simulink model "mvdc_state_estimation"  (R2018b)
settings: configuration reference "Active" (kept outside this file)
undefined symbols (not defined in the file): l_front_m, l_rear_m, P_MLOC_MaxWheelslip_perc, P_MLOC_MaxWheelslipangle_rad, P_MLOC_MinWheelslip_perc, P_MLOC_MinWheelslipangle_rad, P_VDC_ActivateSensorFusion, P_VDC_CurvatureEstimateMax_radpm, P_VDC_CurvatureEstimationMode, P_VDC_LowPassRawSens, P_VDC_LowPassT1Curvature, P_VDC_MinVelSlipCalc_mps, P_VDC_SEResetSamples, tS, TUMStateEstimationState, tw_front_m, tw_rear_m, tyreradius_front_m, tyreradius_rear_m
libraries: simulink x19, misc x3
settings Model: DataDictionary=mvdc_state_estimation.sldd  Creator=wischnewski  LastModifiedBy=ge34qer

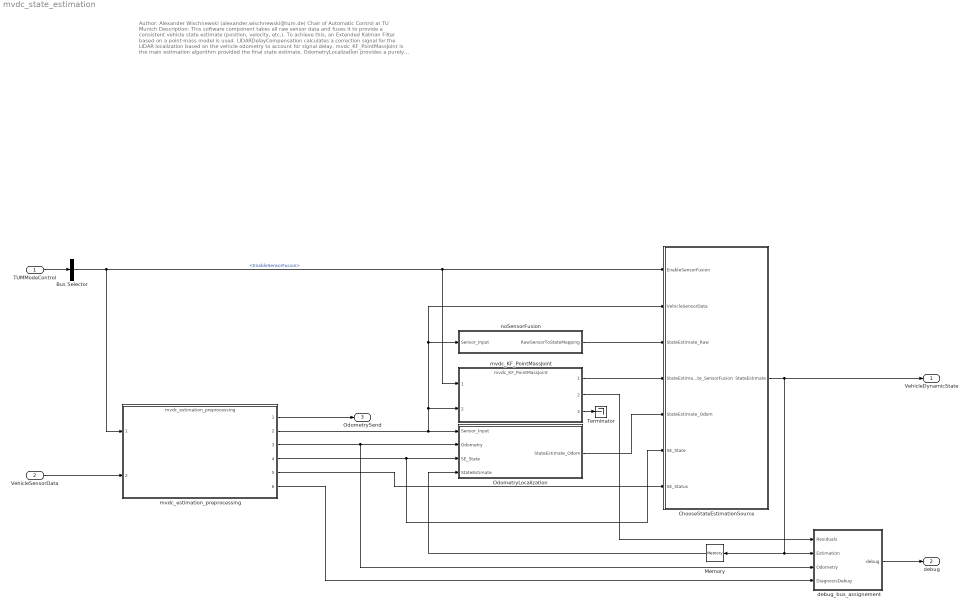
== system mvdc_state_estimation ==
  note: Author: Alexander Wischnewski (alexander.wischnewski@tum.de)
      | Chair of Automatic Control at TU Munich
      |
      | Description: This software component takes all raw sensor data and fuses it to provide a consistent vehicle state estimate (position, velocity, etc.).
      | To achieve this, an Extended Kalman Filter based on a point-mass model is used.
      |
      | LIDARDelayCompensation calculates a correction signal for the LIDAR localization based on the vehicle odometry to account for signal delay.
      |
      | mvdc_KF_PointMassJoint is the main estimation algorithm provided the final state estimate.
      |
      | OdometryLocalization provides a purely odometry based localization based on the last valid position.
      |
      | noSensorFusion provides a bypass solution to the estimator and is used while EnableSensorFusion is not set.
      |
      | mvdc_estimation_preprocessing applies diagnostics on the sensors and generates odometry information.
      |
      | Finally, the debug_bus_assignment forms the debug data.
      |
      | Inputs:
      | TUMModeControl Enable bits which activate the Kalman Filter
      | VehicleSensorData Raw sensor data
      |
      | Outputs:
      | VehicleDynamicState Estimate of the vehicle dynamic state (best available)
      | debug debug data for logging
      | VisualLocSend Data which is send to the LIDAR localization algorithm
  TUMModeControl : Inport  OutDataTypeStr=Bus: TUMModeControl  PortDimensions=1  BusOutputAsStruct=on
  VehicleSensorData : Inport  Port=2  OutDataTypeStr=Bus: VehicleSensorData
  Bus Selector : BusSelector  OutputSignals=EnableSensorFusion
  ChooseStateEstimationSource : Subsystem
  Memory : Memory
  OdometryLocalization : Subsystem
  Terminator : Terminator
  debug_bus_assignement : Subsystem
  mvdc_KF_PointMassJoint : ModelReference  ModelNameDialog=mvdc_KF_PointMassJoint.slx  SimulationMode=Normal  ModelReferenceVersion=1.174
  mvdc_estimation_preprocessing : ModelReference  ModelNameDialog=mvdc_estimation_preprocessing  SimulationMode=Normal  ModelReferenceVersion=1.392
  noSensorFusion : Subsystem
  VehicleDynamicState : Outport  OutDataTypeStr=Bus: VehicleDynamicState
  debug : Outport  Port=2  OutDataTypeStr=Bus: mvdc_state_estimation_debug  PortDimensions=1
  OdometrySend : Outport  Port=3  OutDataTypeStr=Bus: VisualLoc_Send  BusOutputAsStruct=on
  wires:
  mvdc_KF_PointMassJoint/1 -> ChooseStateEstimationSource/4(StateEstimate_SensorFusion)
  Bus Selector/1 -> mvdc_KF_PointMassJoint/1, ChooseStateEstimationSource/1(EnableSensorFusion), mvdc_estimation_preprocessing/1  "<EnableSensorFusion>"
  mvdc_estimation_preprocessing/4 -> ChooseStateEstimationSource/6(SE_State), OdometryLocalization/3(SE_State)
  VehicleSensorData/1 -> mvdc_estimation_preprocessing/2
  mvdc_estimation_preprocessing/2 -> ChooseStateEstimationSource/2(VehicleSensorData), noSensorFusion/1(Sensor_Input), mvdc_KF_PointMassJoint/2, OdometryLocalization/1(Sensor_Input)
  mvdc_estimation_preprocessing/1 -> OdometrySend/1
  ChooseStateEstimationSource/1(StateEstimate) -> Memory/1, debug_bus_assignement/2(Estimation), VehicleDynamicState/1
  mvdc_estimation_preprocessing/3 -> debug_bus_assignement/3(Odometry), OdometryLocalization/2(Odometry)
  OdometryLocalization/1(StateEstimate_Odom) -> ChooseStateEstimationSource/5(StateEstimate_Odom)
  noSensorFusion/1(RawSensorToStateMapping) -> ChooseStateEstimationSource/3(StateEstimate_Raw)
  Memory/1 -> OdometryLocalization/4(StateEstimate)
  debug_bus_assignement/1(debug) -> debug/1
  mvdc_estimation_preprocessing/5 -> ChooseStateEstimationSource/7(SE_Status)
  mvdc_KF_PointMassJoint/2 -> debug_bus_assignement/1(Residuals)
  mvdc_KF_PointMassJoint/3 -> Terminator/1
  TUMModeControl/1 -> Bus Selector/1
  mvdc_estimation_preprocessing/6 -> debug_bus_assignement/4(DiagnosisDebug)

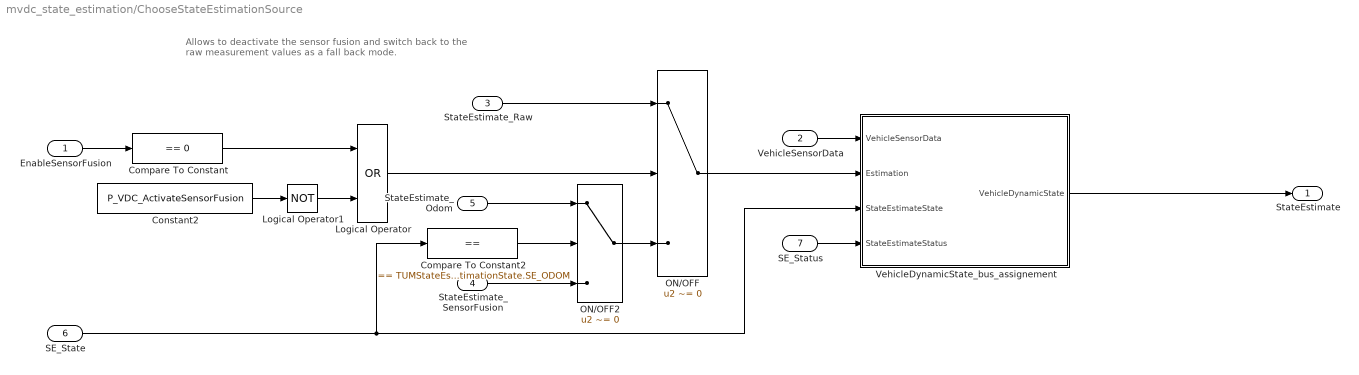
== system mvdc_state_estimation/ChooseStateEstimationSource ==
  note: Allows to deactivate the sensor fusion and switch
      | back to the raw measurement values as a fall back mode.
  EnableSensorFusion : Inport
  VehicleSensorData : Inport  Port=2
  StateEstimate_Raw : Inport  Port=3
  StateEstimate_SensorFusion : Inport  Port=4
  StateEstimate_Odom : Inport  Port=5
  SE_State : Inport  Port=6
  SE_Status : Inport  Port=7
  Compare To Constant : simulink/Logic and Bit Operations/Compare To Constant  relop===  const=0  OutDataTypeStr=boolean
  Compare To Constant2 : simulink/Logic and Bit Operations/Compare To Constant  relop===  const=TUMStateEstimationState.SE_ODOM  OutDataTypeStr=boolean
  Constant2 : Constant  Value=P_VDC_ActivateSensorFusion
  Logical Operator : Logic  Operator=OR  AllPortsSameDT=off  OutDataTypeStr=boolean
  Logical Operator1 : Logic  Operator=NOT  AllPortsSameDT=off  OutDataTypeStr=boolean
  ON/OFF : Switch  Criteria=u2 ~= 0
  ON/OFF2 : Switch  Criteria=u2 ~= 0
  VehicleDynamicState_bus_assignement : Subsystem
  StateEstimate : Outport
  wires:
  StateEstimate_Raw/1 -> ON/OFF/1
  Logical Operator/1 -> ON/OFF/2
  Compare To Constant/1 -> Logical Operator/1
  EnableSensorFusion/1 -> Compare To Constant/1
  SE_State/1 -> VehicleDynamicState_bus_assignement/3(StateEstimateState), Compare To Constant2/1
  ON/OFF/1 -> VehicleDynamicState_bus_assignement/2(Estimation)
  VehicleSensorData/1 -> VehicleDynamicState_bus_assignement/1(VehicleSensorData)
  SE_Status/1 -> VehicleDynamicState_bus_assignement/4(StateEstimateStatus)
  VehicleDynamicState_bus_assignement/1(VehicleDynamicState) -> StateEstimate/1
  ON/OFF2/1 -> ON/OFF/3
  Compare To Constant2/1 -> ON/OFF2/2
  StateEstimate_Odom/1 -> ON/OFF2/1
  StateEstimate_SensorFusion/1 -> ON/OFF2/3
  Constant2/1 -> Logical Operator1/1
  Logical Operator1/1 -> Logical Operator/2

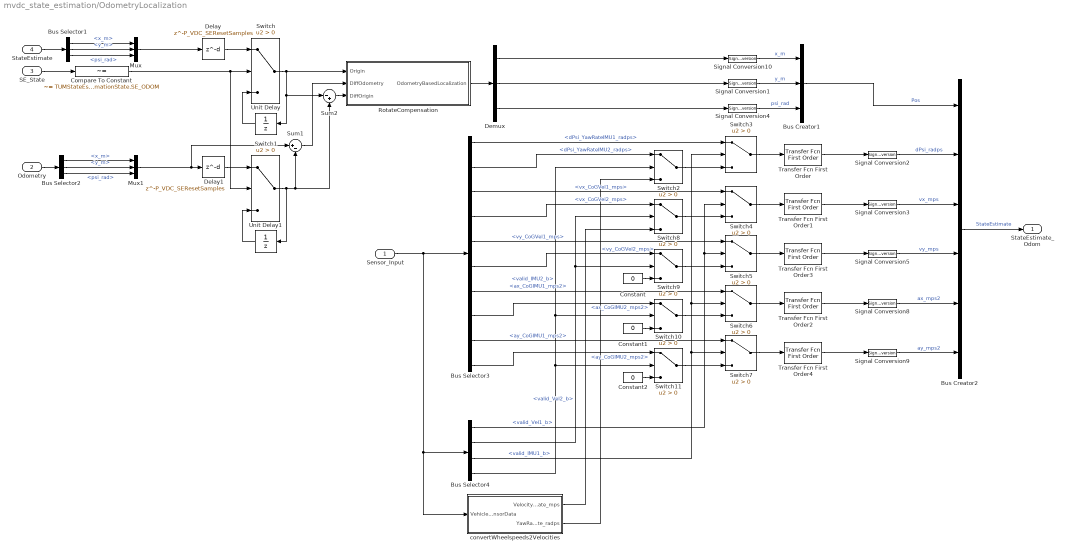
== system mvdc_state_estimation/OdometryLocalization ==
  Sensor_Input : Inport
  Odometry : Inport  Port=2
  SE_State : Inport  Port=3
  StateEstimate : Inport  Port=4
  Bus Creator1 : BusCreator  Inputs=3  OutDataTypeStr=Bus: CartPos
  Bus Creator2 : BusCreator  Inputs=6  OutDataTypeStr=Bus: StateEstimation_state
  Bus Selector1 : BusSelector  OutputSignals=Pos.x_m,Pos.y_m,Pos.psi_rad
  Bus Selector2 : BusSelector  OutputSignals=Position.x_m,Position.y_m,Position.psi_rad
  Bus Selector3 : BusSelector  OutputSignals=dPsi_YawRateIMU1_radps,dPsi_YawRateIMU2_radps,vx_CoGVel1_mps,vx_CoGVel2_mps,vy_CoGVel1_mps,vy_CoGVel2_mps,ax_CoGIMU1_mps2,ax_CoGIMU2_mps2,ay_CoGIMU1_mps2,ay_CoGIMU2_mps2
  Bus Selector4 : BusSelector  OutputSignals=valid_Vel1_b,valid_Vel2_b,valid_IMU1_b,valid_IMU2_b
  Compare To Constant : simulink/Logic and Bit Operations/Compare To Constant  relop=~=  const=TUMStateEstimationState.SE_ODOM  OutDataTypeStr=boolean
  Constant : Constant  Value=0
  Constant1 : Constant  Value=0
  Constant2 : Constant  Value=0
  Delay : Delay  DelayLength=P_VDC_SEResetSamples
  Delay1 : Delay  DelayLength=P_VDC_SEResetSamples
  Demux : Demux  Outputs=3
  Mux : Mux  Inputs=3
  Mux1 : Mux  Inputs=3
  RotateCompensation : Subsystem
  Signal Conversion{1..5,8..10} (8 alike) : SignalConversion  OverrideOpt=off
  Sum1 : Sum  Inputs=|+-
  Sum2 : Sum  Inputs=|-+
  Switch{,1..11} (12 alike) : Switch  Criteria=u2 > Threshold
  Transfer Fcn First Order{,1..4} (5 alike) : simulink/Discrete/Transfer Fcn First Order  PoleZ=exp(-tS/P_VDC_LowPassRawSens)  ICPrevOutput=0.0  DoSatur=off
      settings: SourceProductName=Simulink
  Unit Delay : UnitDelay  SampleTime=-1
  Unit Delay1 : UnitDelay  SampleTime=-1
  convertWheelspeeds2Velocities : Subsystem
  StateEstimate_Odom : Outport
  wires:
  Signal Conversion1/1 -> Bus Creator1/2  "y_m"
  Signal Conversion10/1 -> Bus Creator1/1  "x_m"
  Signal Conversion4/1 -> Bus Creator1/3  "psi_rad"
  Bus Creator2/1 -> StateEstimate_Odom/1  "StateEstimate"
  StateEstimate/1 -> Bus Selector1/1
  Odometry/1 -> Bus Selector2/1
  Delay/1 -> Switch/1
  Unit Delay/1 -> Switch/3
  SE_State/1 -> Compare To Constant/1
  RotateCompensation/1(OdometryBasedLocalization) -> Demux/1
  Demux/1 -> Signal Conversion10/1
  Demux/2 -> Signal Conversion1/1
  Demux/3 -> Signal Conversion4/1
  Switch1/1 -> Sum2/2, Sum1/2, Unit Delay1/1
  Delay1/1 -> Switch1/1
  Unit Delay1/1 -> Switch1/3
  Mux/1 -> Delay/1
  Mux1/1 -> Sum1/1, Delay1/1
  Sum1/1 -> RotateCompensation/2(DIffOdometry)
  Sum2/1 -> RotateCompensation/3(DiffOrigin)
  Switch/1 -> Unit Delay/1, Sum2/1, RotateCompensation/1(Origin)
  Bus Selector1/1 -> Mux/1  "<x_m>"
  Bus Selector1/2 -> Mux/2  "<y_m>"
  Bus Selector1/3 -> Mux/3  "<psi_rad>"
  Bus Selector2/1 -> Mux1/1  "<x_m>"
  Bus Selector2/2 -> Mux1/2  "<y_m>"
  Bus Selector2/3 -> Mux1/3  "<psi_rad>"
  Transfer Fcn First Order2/1 -> Signal Conversion8/1
  Transfer Fcn First Order/1 -> Signal Conversion2/1
  Bus Selector3/7 -> Switch6/1  "<ax_CoGIMU1_mps2>"
  Switch7/1 -> Transfer Fcn First Order4/1
  Transfer Fcn First Order3/1 -> Signal Conversion5/1
  Switch4/1 -> Transfer Fcn First Order1/1
  Transfer Fcn First Order1/1 -> Signal Conversion3/1
  Switch6/1 -> Transfer Fcn First Order2/1
  Bus Selector3/1 -> Switch3/1  "<dPsi_YawRateIMU1_radps>"
  Bus Selector4/3 -> Switch7/2, Switch6/2, Switch3/2  "<valid_IMU1_b>"
  Bus Selector3/9 -> Switch7/1  "<ay_CoGIMU1_mps2>"
  Switch5/1 -> Transfer Fcn First Order3/1
  Bus Selector3/5 -> Switch5/1  "<vy_CoGVel1_mps>"
  Bus Selector3/2 -> Switch2/1  "<dPsi_YawRateIMU2_radps>"
  Signal Conversion8/1 -> Bus Creator2/5  "ax_mps2"
  Signal Conversion2/1 -> Bus Creator2/2  "dPsi_radps"
  Signal Conversion3/1 -> Bus Creator2/3  "vx_mps"
  Switch3/1 -> Transfer Fcn First Order/1
  Signal Conversion9/1 -> Bus Creator2/6  "ay_mps2"
  Sensor_Input/1 -> convertWheelspeeds2Velocities/1(VehicleSensorData), Bus Selector4/1, Bus Selector3/1
  Signal Conversion5/1 -> Bus Creator2/4  "vy_mps"
  Bus Selector4/1 -> Switch5/2, Switch4/2  "<valid_Vel1_b>"
  Bus Selector3/3 -> Switch4/1  "<vx_CoGVel1_mps>"
  Transfer Fcn First Order4/1 -> Signal Conversion9/1
  Bus Selector4/4 -> Switch11/2, Switch10/2, Switch2/2  "<valid_IMU2_b>"
  Bus Selector4/2 -> Switch9/2, Switch8/2  "<valid_Vel2_b>"
  Bus Creator1/1 -> Bus Creator2/1  "Pos"
  Compare To Constant/1 -> Switch1/2, Switch/2
  Switch2/1 -> Switch3/3
  convertWheelspeeds2Velocities/2(YawRateEstimate_radps) -> Switch2/3
  Switch8/1 -> Switch4/3
  Bus Selector3/4 -> Switch8/1  "<vx_CoGVel2_mps>"
  convertWheelspeeds2Velocities/1(VelocityEstimate_mps) -> Switch8/3
  Switch9/1 -> Switch5/3
  Bus Selector3/6 -> Switch9/1  "<vy_CoGVel2_mps>"
  Constant/1 -> Switch9/3
  Switch10/1 -> Switch6/3
  Bus Selector3/8 -> Switch10/1  "<ax_CoGIMU2_mps2>"
  Constant1/1 -> Switch10/3
  Switch11/1 -> Switch7/3
  Bus Selector3/10 -> Switch11/1  "<ay_CoGIMU2_mps2>"
  Constant2/1 -> Switch11/3

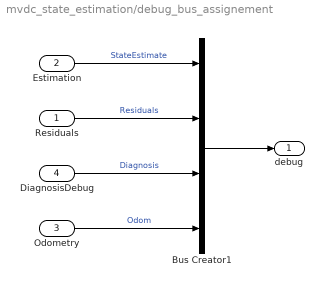
== system mvdc_state_estimation/debug_bus_assignement ==
  Residuals : Inport
  Estimation : Inport  Port=2
  Odometry : Inport  Port=3
  DiagnosisDebug : Inport  Port=4
  Bus Creator1 : BusCreator  Inputs=4
  debug : Outport
  wires:
  Bus Creator1/1 -> debug/1
  Estimation/1 -> Bus Creator1/1  "StateEstimate"
  Residuals/1 -> Bus Creator1/2  "Residuals"
  DiagnosisDebug/1 -> Bus Creator1/3  "Diagnosis"
  Odometry/1 -> Bus Creator1/4  "Odom"

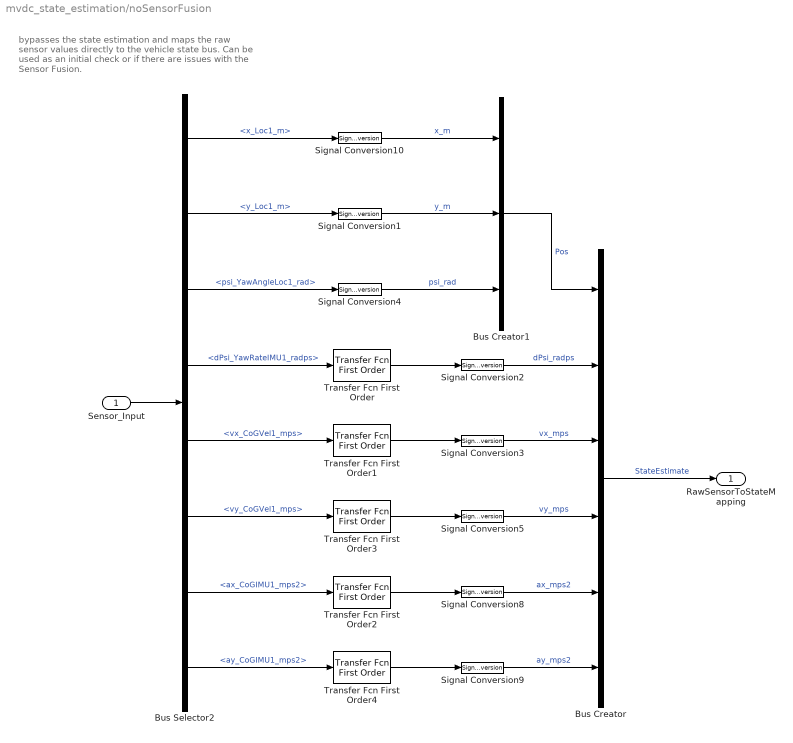
== system mvdc_state_estimation/noSensorFusion ==
  note: bypasses the state estimation and maps the
      | raw sensor values directly to the vehicle state bus.
      | Can be used as an initial check or if there are
      | issues with the Sensor Fusion.
  Sensor_Input : Inport
  Bus Creator : BusCreator  Inputs=6  OutDataTypeStr=Bus: StateEstimation_state
  Bus Creator1 : BusCreator  Inputs=3  OutDataTypeStr=Bus: CartPos
  Bus Selector2 : BusSelector  OutputSignals=x_Loc1_m,y_Loc1_m,psi_YawAngleLoc1_rad,dPsi_YawRateIMU1_radps,vx_CoGVel1_mps,vy_CoGVel1_mps,ax_CoGIMU1_mps2,ay_CoGIMU1_mps2
  Signal Conversion{1..5,8..10} (8 alike) : SignalConversion  OverrideOpt=off
  Transfer Fcn First Order{,1..4} (5 alike) : simulink/Discrete/Transfer Fcn First Order  PoleZ=exp(-tS/P_VDC_LowPassRawSens)  ICPrevOutput=0.0  DoSatur=off
      settings: SourceProductName=Simulink
  RawSensorToStateMapping : Outport
  wires:
  Sensor_Input/1 -> Bus Selector2/1
  Bus Creator1/1 -> Bus Creator/1  "Pos"
  Signal Conversion4/1 -> Bus Creator1/3  "psi_rad"
  Signal Conversion2/1 -> Bus Creator/2  "dPsi_radps"
  Signal Conversion3/1 -> Bus Creator/3  "vx_mps"
  Signal Conversion5/1 -> Bus Creator/4  "vy_mps"
  Signal Conversion8/1 -> Bus Creator/5  "ax_mps2"
  Signal Conversion9/1 -> Bus Creator/6  "ay_mps2"
  Bus Creator/1 -> RawSensorToStateMapping/1  "StateEstimate"
  Signal Conversion1/1 -> Bus Creator1/2  "y_m"
  Signal Conversion10/1 -> Bus Creator1/1  "x_m"
  Bus Selector2/7 -> Transfer Fcn First Order2/1  "<ax_CoGIMU1_mps2>"
  Bus Selector2/8 -> Transfer Fcn First Order4/1  "<ay_CoGIMU1_mps2>"
  Bus Selector2/6 -> Transfer Fcn First Order3/1  "<vy_CoGVel1_mps>"
  Bus Selector2/4 -> Transfer Fcn First Order/1  "<dPsi_YawRateIMU1_radps>"
  Bus Selector2/5 -> Transfer Fcn First Order1/1  "<vx_CoGVel1_mps>"
  Bus Selector2/1 -> Signal Conversion10/1  "<x_Loc1_m>"
  Bus Selector2/2 -> Signal Conversion1/1  "<y_Loc1_m>"
  Bus Selector2/3 -> Signal Conversion4/1  "<psi_YawAngleLoc1_rad>"
  Transfer Fcn First Order3/1 -> Signal Conversion5/1
  Transfer Fcn First Order1/1 -> Signal Conversion3/1
  Transfer Fcn First Order/1 -> Signal Conversion2/1
  Transfer Fcn First Order4/1 -> Signal Conversion9/1
  Transfer Fcn First Order2/1 -> Signal Conversion8/1

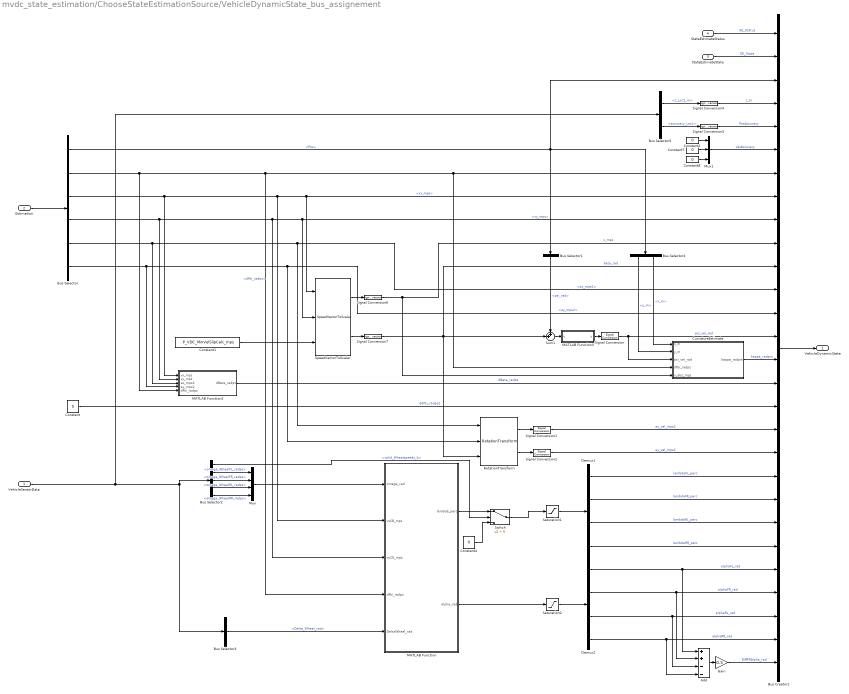
== system mvdc_state_estimation/ChooseStateEstimationSource/VehicleDynamicState_bus_assignement ==
  VehicleSensorData : Inport
  Estimation : Inport  Port=2
  StateEstimateState : Inport  Port=3  OutDataTypeStr=Enum: TUMStateEstimationState  BusOutputAsStruct=on
  StateEstimateStatus : Inport  Port=4  OutDataTypeStr=Enum: TUMHealthStatus  BusOutputAsStruct=on
  Add : Sum  Inputs=++--
  Bus Creator1 : BusCreator  Inputs=28
  Bus Selector : BusSelector  OutputSignals=Pos,dPsi_radps,vx_mps,vy_mps,ax_mps2,ay_mps2
  Bus Selector1 : BusSelector  OutputSignals=psi_rad
  Bus Selector2 : BusSelector  OutputSignals=valid_Wheelspeeds_b,omega_WheelFL_radps,omega_WheelFR_radps,omega_WheelRL_radps,omega_WheelRR_radps
  Bus Selector3 : BusSelector  OutputSignals=Delta_Wheel_rad
  Bus Selector4 : BusSelector  OutputSignals=y_m,x_m
  Bus Selector5 : BusSelector  OutputSignals=z_Loc1_m,accuracy_Loc1
  Constant{,2,4,7..8} (5 alike) : Constant  Value=0
  Constant1 : Constant  Value=P_VDC_MinVelSlipCalc_mps
  CurvatureEstimate : Subsystem
  Demux1 : Demux
  Demux2 : Demux
  Gain : Gain  Gain=0.5
  MATLAB Function : MATLAB Function  TreatAsAtomicUnit=on
  MATLAB Function2 : MATLAB Function  TreatAsAtomicUnit=on
  MATLAB Function3 : MATLAB Function  TreatAsAtomicUnit=on
  Mux : Mux
  Mux1 : Mux  Inputs=3
  RotationTransform : misc/RotationTransform  SystemSampleTime=-1
  Saturation1 : Saturate  UpperLimit=P_MLOC_MaxWheelslip_perc  LowerLimit=P_MLOC_MinWheelslip_perc
  Saturation2 : Saturate  UpperLimit=P_MLOC_MaxWheelslipangle_rad  LowerLimit=P_MLOC_MinWheelslipangle_rad
  Signal Conversion{,1..4,6..7} (7 alike) : SignalConversion  OverrideOpt=off
  SpeedVectorToScalar : misc/SpeedVectorToScalar  SystemSampleTime=-1
  Sum1 : Sum  Inputs=++|
  Switch : Switch  Criteria=u2 > Threshold
  VehicleDynamicState : Outport
  wires:
  Bus Creator1/1 -> VehicleDynamicState/1
  Sum1/1 -> MATLAB Function3/1(u)
  Bus Selector/3 -> MATLAB Function2/1(vx_mps), MATLAB Function/2(vxCB_mps), SpeedVectorToScalar/1, Bus Creator1/8  "<vx_mps>"
  Bus Selector/1 -> Bus Selector4/1, Bus Creator1/3, Bus Selector1/1  "<Pos>"
  Bus Selector1/1 -> Sum1/1  "<psi_rad>"
  Estimation/1 -> Bus Selector/1
  StateEstimateState/1 -> Bus Creator1/2  "SE_State"
  MATLAB Function3/1(y) -> Signal Conversion/1
  CurvatureEstimate/1(kappa_radpm) -> Bus Creator1/15  "kappa_radpm"
  Signal Conversion/1 -> Bus Creator1/14, CurvatureEstimate/3(psi_vel_rad)  "psi_vel_rad"
  MATLAB Function2/1(dBeta_radps) -> Bus Creator1/16  "dBeta_radps"
  Constant/1 -> Bus Creator1/17  "ddPsi_radps2"
  Bus Selector/4 -> MATLAB Function/3(vyCG_mps), Bus Creator1/9, SpeedVectorToScalar/2, MATLAB Function2/2(vy_mps)  "<vy_mps>"
  SpeedVectorToScalar/1 -> Signal Conversion6/1
  SpeedVectorToScalar/2 -> Signal Conversion7/1
  Signal Conversion6/1 -> Bus Creator1/10, CurvatureEstimate/5(v_abs_mps)  "v_mps"
  Bus Selector/5 -> MATLAB Function2/3(ax_mps2), RotationTransform/1, Bus Creator1/12  "<ax_mps2>"
  Bus Selector/6 -> RotationTransform/2, Bus Creator1/13, MATLAB Function2/4(ay_mps2)  "<ay_mps2>"
  Signal Conversion7/1 -> Sum1/2, RotationTransform/3, Bus Creator1/11  "beta_rad"
  RotationTransform/1 -> Signal Conversion1/1
  RotationTransform/2 -> Signal Conversion2/1
  Signal Conversion1/1 -> Bus Creator1/18  "ax_vel_mps2"
  Signal Conversion2/1 -> Bus Creator1/19  "ay_vel_mps2"
  Bus Selector/2 -> MATLAB Function2/5(dPsi_radps), MATLAB Function/4(dPsi_radps), Bus Creator1/7, CurvatureEstimate/4(dPsi_radps)  "<dPsi_radps>"
  Saturation1/1 -> Demux1/1
  Saturation2/1 -> Demux2/1
  Demux2/1 -> Bus Creator1/24, Add/1  "alphaFL_rad"
  Demux2/2 -> Bus Creator1/25, Add/2  "alphaFR_rad"
  Demux2/3 -> Bus Creator1/26, Add/3  "alphaRL_rad"
  Demux2/4 -> Bus Creator1/27, Add/4  "alphaRR_rad"
  Demux1/1 -> Bus Creator1/20  "lambdaFL_perc"
  Demux1/2 -> Bus Creator1/21  "lambdaFR_perc"
  Demux1/3 -> Bus Creator1/22  "lambdaRL_perc"
  Demux1/4 -> Bus Creator1/23  "lambdaRR_perc"
  VehicleSensorData/1 -> Bus Selector5/1, Bus Selector3/1, Bus Selector2/1
  Bus Selector2/2 -> Mux/1  "<omega_WheelFL_radps>"
  Bus Selector2/3 -> Mux/2  "<omega_WheelFR_radps>"
  Bus Selector2/4 -> Mux/3  "<omega_WheelRL_radps>"
  Bus Selector2/5 -> Mux/4  "<omega_WheelRR_radps>"
  Mux/1 -> MATLAB Function/1(omega_rad)
  Bus Selector3/1 -> MATLAB Function/5(DeltaWheel_rad)  "<Delta_Wheel_rad>"
  Constant1/1 -> SpeedVectorToScalar/3
  Bus Selector4/1 -> CurvatureEstimate/2(y_m)  "<y_m>"
  Bus Selector4/2 -> CurvatureEstimate/1("x_m ")  "<x_m>"
  Bus Selector5/2 -> Signal Conversion3/1  "<accuracy_Loc1>"
  Constant8/1 -> Mux1/3
  Mux1/1 -> Bus Creator1/6  "VelAccuracy"
  Constant2/1 -> Mux1/1
  Constant7/1 -> Mux1/2
  Signal Conversion3/1 -> Bus Creator1/5  "PosAccuracy"
  Bus Selector5/1 -> Signal Conversion4/1  "<z_Loc1_m>"
  Signal Conversion4/1 -> Bus Creator1/4  "z_m"
  StateEstimateStatus/1 -> Bus Creator1/1  "SE_Status"
  MATLAB Function/1(lambda_perc) -> Switch/1
  Switch/1 -> Saturation1/1
  MATLAB Function/2(alpha_rad) -> Saturation2/1
  Bus Selector2/1 -> Switch/2  "<valid_Wheelspeeds_b>"
  Constant4/1 -> Switch/3
  Add/1 -> Gain/1
  Gain/1 -> Bus Creator1/28  "DiffFRAlpha_rad"

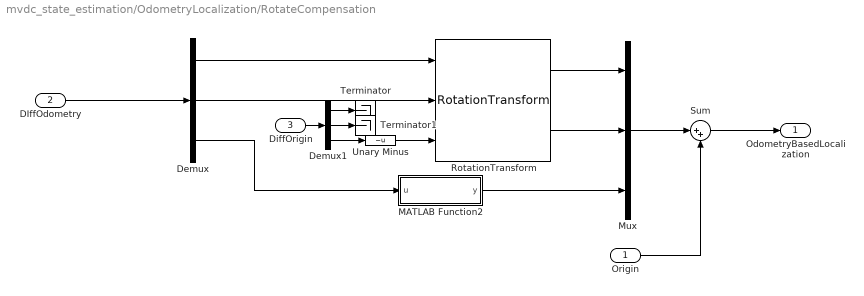
== system mvdc_state_estimation/OdometryLocalization/RotateCompensation ==
  Origin : Inport
  DIffOdometry : Inport  Port=2
  DiffOrigin : Inport  Port=3
  Demux : Demux  Outputs=3
  Demux1 : Demux  Outputs=3
  MATLAB Function2 : MATLAB Function  TreatAsAtomicUnit=on
  Mux : Mux  Inputs=3
  RotationTransform : misc/RotationTransform  SystemSampleTime=-1
  Sum : Sum  Inputs=|++
  Terminator : Terminator
  Terminator1 : Terminator
  Unary Minus : UnaryMinus
  OdometryBasedLocalization : Outport
  wires:
  Demux/3 -> MATLAB Function2/1(u)
  RotationTransform/1 -> Mux/1
  RotationTransform/2 -> Mux/2
  MATLAB Function2/1(y) -> Mux/3
  Demux/2 -> RotationTransform/2
  Demux/1 -> RotationTransform/1
  DIffOdometry/1 -> Demux/1
  Mux/1 -> Sum/1
  Sum/1 -> OdometryBasedLocalization/1
  Origin/1 -> Sum/2
  DiffOrigin/1 -> Demux1/1
  Demux1/3 -> Unary Minus/1
  Demux1/1 -> Terminator/1
  Demux1/2 -> Terminator1/1
  Unary Minus/1 -> RotationTransform/3

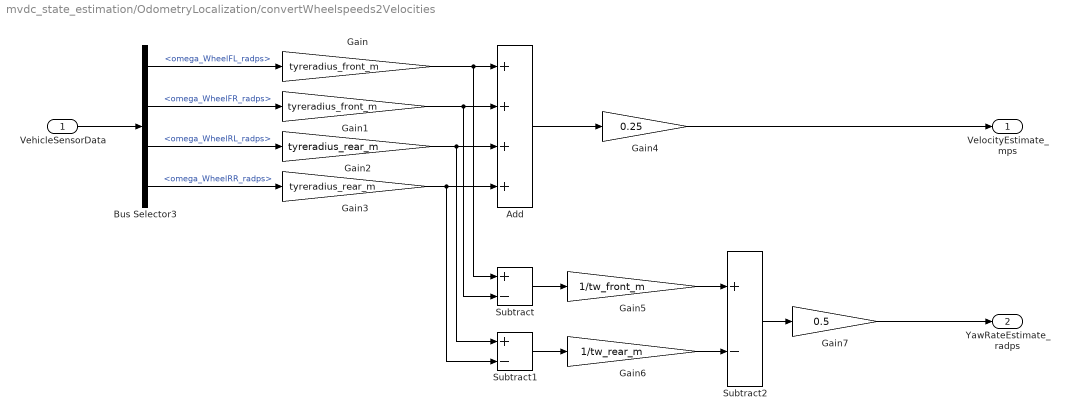
== system mvdc_state_estimation/OdometryLocalization/convertWheelspeeds2Velocities ==
  VehicleSensorData : Inport
  Add : Sum  Inputs=4
  Bus Selector3 : BusSelector  OutputSignals=omega_WheelFL_radps,omega_WheelFR_radps,omega_WheelRL_radps,omega_WheelRR_radps
  Gain : Gain  Gain=tyreradius_front_m
  Gain1 : Gain  Gain=tyreradius_front_m
  Gain2 : Gain  Gain=tyreradius_rear_m
  Gain3 : Gain  Gain=tyreradius_rear_m
  Gain4 : Gain  Gain=0.25
  Gain5 : Gain  Gain=1/tw_front_m
  Gain6 : Gain  Gain=1/tw_rear_m
  Gain7 : Gain  Gain=0.5
  Subtract : Sum  Inputs=+-
  Subtract1 : Sum  Inputs=+-
  Subtract2 : Sum  Inputs=+-
  VelocityEstimate_mps : Outport
  YawRateEstimate_radps : Outport  Port=2
  wires:
  Gain2/1 -> Subtract1/1, Add/3
  Gain/1 -> Subtract/1, Add/1
  Bus Selector3/3 -> Gain2/1  "<omega_WheelRL_radps>"
  VehicleSensorData/1 -> Bus Selector3/1
  Gain1/1 -> Subtract/2, Add/2
  Bus Selector3/4 -> Gain3/1  "<omega_WheelRR_radps>"
  Bus Selector3/1 -> Gain/1  "<omega_WheelFL_radps>"
  Bus Selector3/2 -> Gain1/1  "<omega_WheelFR_radps>"
  Gain3/1 -> Subtract1/2, Add/4
  Add/1 -> Gain4/1
  Gain4/1 -> VelocityEstimate_mps/1
  Subtract/1 -> Gain5/1
  Subtract1/1 -> Gain6/1
  Gain5/1 -> Subtract2/1
  Gain6/1 -> Subtract2/2
  Subtract2/1 -> Gain7/1
  Gain7/1 -> YawRateEstimate_radps/1

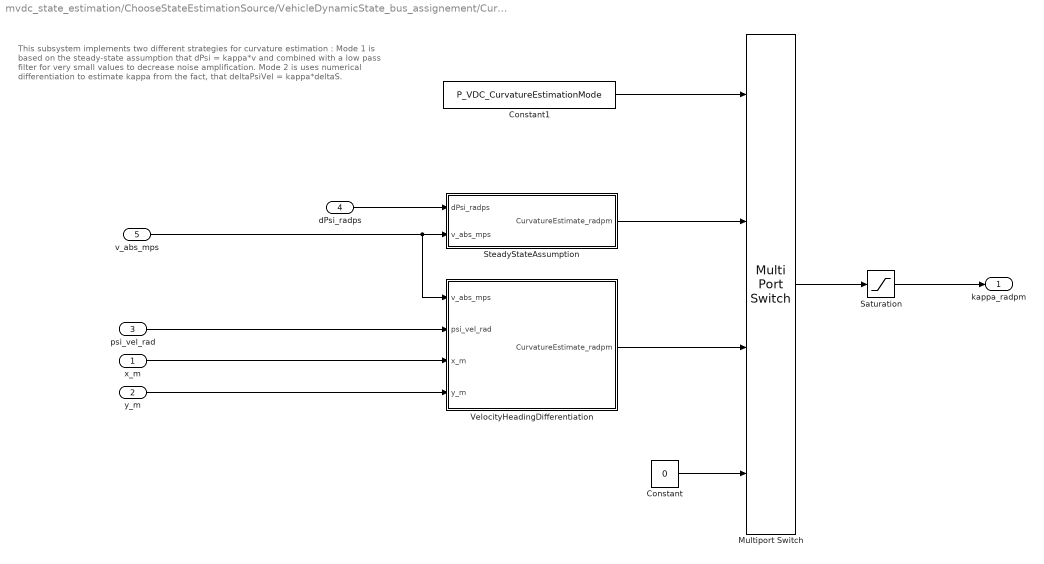
== system mvdc_state_estimation/ChooseStateEstimationSource/VehicleDynamicState_bus_assignement/CurvatureEstimate ==
  note: This subsystem implements two different strategies for curvature estimation :
      |
      | Mode 1 is based on the steady-state assumption that dPsi = kappa*v and combined
      | with a low pass filter for very small values to decrease noise amplification.
      |
      | Mode 2 is uses numerical differentiation to estimate kappa from the fact, that
      | deltaPsiVel = kappa*deltaS.
  "x_m " : Inport
  y_m : Inport  Port=2
  psi_vel_rad : Inport  Port=3
  dPsi_radps : Inport  Port=4
  v_abs_mps : Inport  Port=5
  Constant : Constant  Value=0
  Constant1 : Constant  Value=P_VDC_CurvatureEstimationMode
  Multiport Switch : MultiPortSwitch  Inputs=2  DataPortForDefault=Additional data port
  Saturation : Saturate  UpperLimit=P_VDC_CurvatureEstimateMax_radpm  LowerLimit=-P_VDC_CurvatureEstimateMax_radpm
  SteadyStateAssumption : Subsystem
  VelocityHeadingDifferentiation : Subsystem
  kappa_radpm : Outport
  wires:
  Constant/1 -> Multiport Switch/4
  dPsi_radps/1 -> SteadyStateAssumption/1(dPsi_radps)
  SteadyStateAssumption/1(CurvatureEstimate_radpm) -> Multiport Switch/2
  v_abs_mps/1 -> VelocityHeadingDifferentiation/1(v_abs_mps), SteadyStateAssumption/2(v_abs_mps)
  psi_vel_rad/1 -> VelocityHeadingDifferentiation/2(psi_vel_rad)
  "x_m "/1 -> VelocityHeadingDifferentiation/3("x_m ")
  y_m/1 -> VelocityHeadingDifferentiation/4(y_m)
  VelocityHeadingDifferentiation/1(CurvatureEstimate_radpm) -> Multiport Switch/3
  Constant1/1 -> Multiport Switch/1
  Multiport Switch/1 -> Saturation/1
  Saturation/1 -> kappa_radpm/1

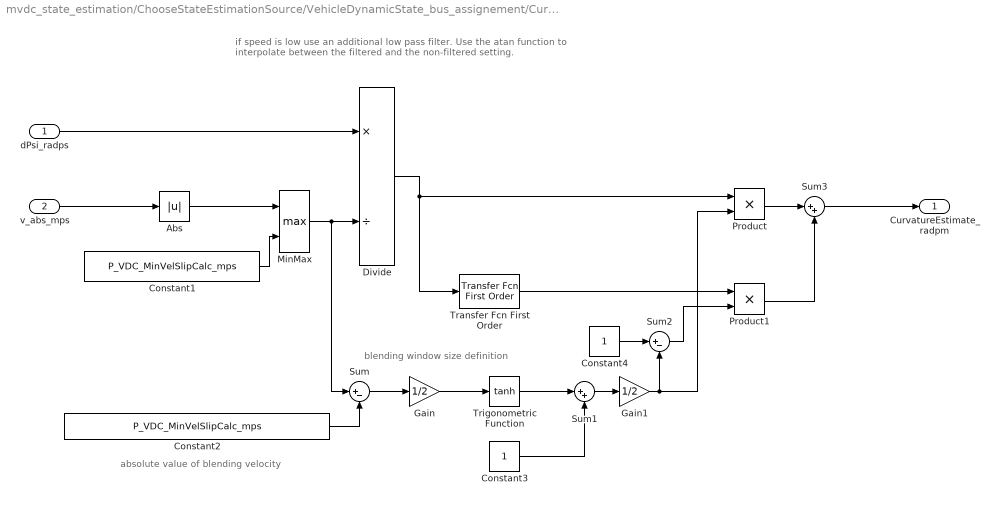
== system mvdc_state_estimation/ChooseStateEstimationSource/VehicleDynamicState_bus_assignement/CurvatureEstimate/SteadyStateAssumption ==
  note: blending window size definition
  note: absolute value of blending velocity
  note: if speed is low use an additional low pass filter.
      | Use the atan function to interpolate between the filtered and the non-filtered setting.
  dPsi_radps : Inport
  v_abs_mps : Inport  Port=2
  Abs : Abs
  Constant1 : Constant  Value=P_VDC_MinVelSlipCalc_mps
  Constant2 : Constant  Value=P_VDC_MinVelSlipCalc_mps
  Constant3 : Constant
  Constant4 : Constant
  Divide : Product  Inputs=*/
  Gain : Gain  Gain=1/2
  Gain1 : Gain  Gain=1/2
  MinMax : MinMax  Function=max  Inputs=2
  Product : Product
  Product1 : Product
  Sum : Sum  Inputs=|+-
  Sum1 : Sum  Inputs=|++
  Sum2 : Sum  Inputs=|+-
  Sum3 : Sum  Inputs=|++
  Transfer Fcn First Order : simulink/Discrete/Transfer Fcn First Order  PoleZ=exp(-tS/P_VDC_LowPassT1Curvature)  ICPrevOutput=0.0  DoSatur=off
      settings: SourceProductName=Simulink
  Trigonometric Function : Trigonometry  Operator=tanh
  CurvatureEstimate_radpm : Outport
  wires:
  Sum/1 -> Gain/1
  MinMax/1 -> Sum/1, Divide/2
  Constant1/1 -> MinMax/2
  Constant3/1 -> Sum1/2
  Divide/1 -> Transfer Fcn First Order/1, Product/1
  Constant4/1 -> Sum2/1
  Trigonometric Function/1 -> Sum1/1
  Gain/1 -> Trigonometric Function/1
  Constant2/1 -> Sum/2
  Abs/1 -> MinMax/1
  Product1/1 -> Sum3/2
  Sum1/1 -> Gain1/1
  Gain1/1 -> Product/2, Sum2/2
  Product/1 -> Sum3/1
  Sum2/1 -> Product1/2
  Transfer Fcn First Order/1 -> Product1/1
  v_abs_mps/1 -> Abs/1
  dPsi_radps/1 -> Divide/1
  Sum3/1 -> CurvatureEstimate_radpm/1

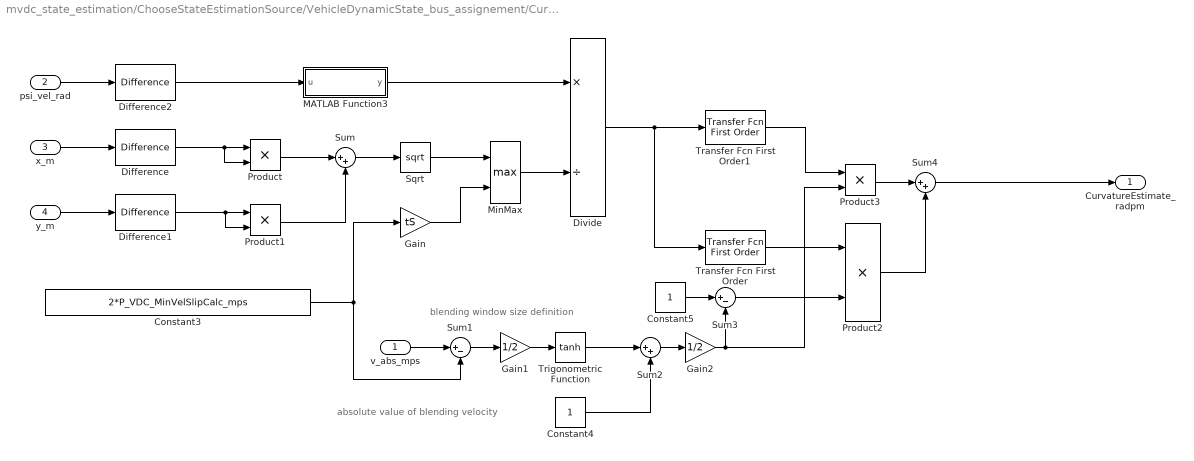
== system mvdc_state_estimation/ChooseStateEstimationSource/VehicleDynamicState_bus_assignement/CurvatureEstimate/VelocityHeadingDifferentiation ==
  note: absolute value of blending velocity
  note: blending window size definition
  v_abs_mps : Inport
  psi_vel_rad : Inport  Port=2
  "x_m " : Inport  Port=3
  y_m : Inport  Port=4
  Constant3 : Constant  Value=2*P_VDC_MinVelSlipCalc_mps
  Constant4 : Constant
  Constant5 : Constant
  Difference : simulink/Discrete/Difference  ICPrevInput=0.0  OutMin=[]  OutMax=[]  OutDataType=fixdt(1, 16)  OutScaling=2^-10  DoSatur=off
  Difference1 : simulink/Discrete/Difference  ICPrevInput=0.0  OutMin=[]  OutMax=[]  OutDataType=fixdt(1, 16)  OutScaling=2^-10  DoSatur=off
  Difference2 : simulink/Discrete/Difference  ICPrevInput=0.0  OutMin=[]  OutMax=[]  OutDataType=fixdt(1, 16)  OutScaling=2^-10  DoSatur=off
  Divide : Product  Inputs=*/
  Gain : Gain  Gain=tS
  Gain1 : Gain  Gain=1/2
  Gain2 : Gain  Gain=1/2
  MATLAB Function3 : MATLAB Function  TreatAsAtomicUnit=on
  MinMax : MinMax  Function=max  Inputs=2
  Product{,1..3} (4 alike) : Product
  Sqrt : Sqrt  SaturateOnIntegerOverflow=on
  Sum : Sum  Inputs=|++
  Sum1 : Sum  Inputs=|+-
  Sum2 : Sum  Inputs=|++
  Sum3 : Sum  Inputs=|+-
  Sum4 : Sum  Inputs=|++
  Transfer Fcn First Order : simulink/Discrete/Transfer Fcn First Order  PoleZ=exp(-tS/P_VDC_LowPassT1Curvature)  ICPrevOutput=0.0  DoSatur=off
      settings: SourceProductName=Simulink
  Transfer Fcn First Order1 : simulink/Discrete/Transfer Fcn First Order  PoleZ=exp(-tS/(0.5*P_VDC_LowPassT1Curvature))  ICPrevOutput=0.0  DoSatur=off
      settings: SourceProductName=Simulink
  Trigonometric Function : Trigonometry  Operator=tanh
  CurvatureEstimate_radpm : Outport
  wires:
  Difference1/1 -> Product1/2, Product1/1
  Difference/1 -> Product/2, Product/1
  Product1/1 -> Sum/2
  Transfer Fcn First Order/1 -> Product2/1
  Product/1 -> Sum/1
  MinMax/1 -> Divide/2
  Constant4/1 -> Sum2/2
  Difference2/1 -> MATLAB Function3/1(u)
  Sum2/1 -> Gain2/1
  Gain/1 -> MinMax/2
  Sum/1 -> Sqrt/1
  Constant3/1 -> Sum1/2, Gain/1
  Product2/1 -> Sum4/2
  y_m/1 -> Difference1/1
  "x_m "/1 -> Difference/1
  Sum3/1 -> Product2/2
  Gain1/1 -> Trigonometric Function/1
  Gain2/1 -> Product3/2, Sum3/2
  Constant5/1 -> Sum3/1
  v_abs_mps/1 -> Sum1/1
  psi_vel_rad/1 -> Difference2/1
  Trigonometric Function/1 -> Sum2/1
  Sum1/1 -> Gain1/1
  Sqrt/1 -> MinMax/1
  Product3/1 -> Sum4/1
  Divide/1 -> Transfer Fcn First Order/1, Transfer Fcn First Order1/1
  Sum4/1 -> CurvatureEstimate_radpm/1
  MATLAB Function3/1(y) -> Divide/1
  Transfer Fcn First Order1/1 -> Product3/1

== matlab function mvdc_state_estimation/ChooseStateEstimationSource/VehicleDynamicState_bus_assignement/CurvatureEstimate/VelocityHeadingDifferentiation/MATLAB Function3 ==
  data: u input; y output
function y = fcn(u)

y = normalizeAngle(u);

== matlab function mvdc_state_estimation/OdometryLocalization/RotateCompensation/MATLAB Function2 ==
  data: u input; y output
function y = fcn(u)

y = normalizeAngle(u);

== matlab function mvdc_state_estimation/ChooseStateEstimationSource/VehicleDynamicState_bus_assignement/MATLAB Function ==
  data: omega_rad input size=4; vxCB_mps input; vyCG_mps input; dPsi_radps input; DeltaWheel_rad input; lambda_perc output; alpha_rad output; tyreradius_rear_m parameter; tyreradius_front_m parameter; tw_rear_m parameter; tw_front_m parameter; l_rear_m parameter; l_front_m parameter; P_VDC_MinVelSlipCalc_mps parameter
function [lambda_perc, alpha_rad] = fcn(omega_rad, vxCB_mps, vyCG_mps, dPsi_radps, DeltaWheel_rad, tyreradius_rear_m, tyreradius_front_m, tw_rear_m, tw_front_m, l_rear_m, l_front_m, P_VDC_MinVelSlipCalc_mps)
%#codegen
  [lambda_perc, alpha_rad] = calcWheelSlips(omega_rad, [vxCB_mps; vyCG_mps; dPsi_radps], DeltaWheel_rad, tw_front_m, tw_rear_m, l_front_m, l_rear_m, tyreradius_front_m, tyreradius_rear_m, P_VDC_MinVelSlipCalc_mps);

== matlab function mvdc_state_estimation/ChooseStateEstimationSource/VehicleDynamicState_bus_assignement/MATLAB Function2 ==
  data: vx_mps input; dBeta_radps output; vy_mps input; ax_mps2 input; ay_mps2 input; dPsi_radps input
function dBeta_radps = fcn(vx_mps, vy_mps, ax_mps2, ay_mps2, dPsi_radps )
%#codegen

[ dBeta_radps ] = calc_dBeta( vx_mps, vy_mps, ax_mps2, ay_mps2, dPsi_radps );

== matlab function mvdc_state_estimation/ChooseStateEstimationSource/VehicleDynamicState_bus_assignement/MATLAB Function3 ==
  data: u input; y output
function y = fcn(u)

y = normalizeAngle(u);
